simulink model "untitled5"  (R2019b)
settings: Solver=VariableStepAuto  StartTime=0.0  StopTime=60  RelTol=1e-3
model workspace (MAT data in the model file):
  A = Simulink.Signal
  A.DataType = 'double'
  A.Min = 0
  A.Dimensions = 1
  A.DimensionsMode = 'auto'
  A.Complexity = 'auto'
  A.SampleTime = -1
  A.SamplingMode = 'auto'
  A.InitialValue = '0'
values from neighbouring files (symbols this model uses):
  Brad = 0.17    [lab5.m]
  J = 0.0023    [lab5.m]
  Ke = Km    (= 0.29)    [lab5.m]
  Km = 0.29    [lab5.m]
  Kr = 70    [lab5.m]
  Ks = 250    [lab5.m]
  L = 0.0047    [lab5.m]
  R = 4.7    [lab5.m]
  Rad = 0.0275    [lab5.m]
  Um = 3.5    [lab5.m]
settings Model: Creator=Ivan  LastModifiedBy=Ivan
settings SolverCC: AlgebraicLoopSolver=LineSearch

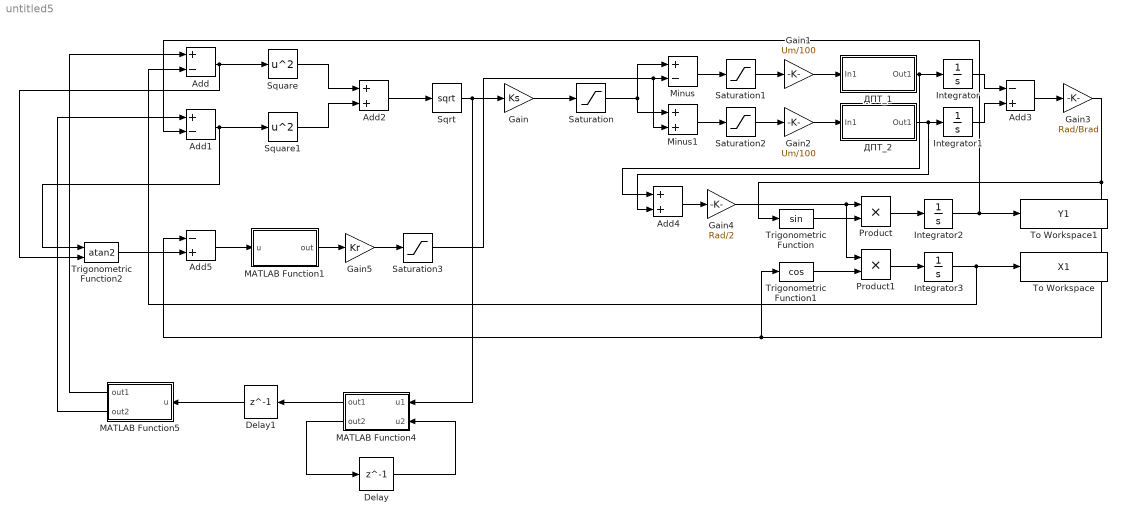
== system untitled5 ==
  Add : Sum  Inputs=+-
  Add1 : Sum  Inputs=+-
  Add2 : Sum
  Add3 : Sum  Inputs=-+
  Add4 : Sum
  Add5 : Sum  Inputs=-+
  Delay : Delay  DelayLength=1  InitialCondition=0
  Delay1 : Delay  DelayLength=1  InitialCondition=0
  Gain : Gain  Gain=Ks
  Gain1 : Gain  Gain=Um/100
  Gain2 : Gain  Gain=Um/100
  Gain3 : Gain  Gain=Rad/Brad
  Gain4 : Gain  Gain=Rad/2
  Gain5 : Gain  Gain=Kr
  Integrator{,1..3} (4 alike) : Integrator
  MATLAB Function1 : MATLAB Function  TreatAsAtomicUnit=on  VariantControl=Variant1
  MATLAB Function4 : MATLAB Function  TreatAsAtomicUnit=on  VariantControl=Variant1
  MATLAB Function5 : MATLAB Function  TreatAsAtomicUnit=on  VariantControl=Variant1
  Minus : Sum  Inputs=+-
  Minus1 : Sum
  Product : Product
  Product1 : Product
  Saturation : Saturate  UpperLimit=80  LowerLimit=-80
  Saturation1 : Saturate  UpperLimit=100  LowerLimit=-100
  Saturation2 : Saturate  UpperLimit=100  LowerLimit=-100
  Saturation3 : Saturate  UpperLimit=20  LowerLimit=-20
  Sqrt : Sqrt  SaturateOnIntegerOverflow=on
  Square : Math  Operator=square  SignedPower=off  SaturateOnIntegerOverflow=on
  Square1 : Math  Operator=square  SignedPower=off  SaturateOnIntegerOverflow=on
  To Workspace : ToWorkspace  VariableName=X1  SaveFormat=Timeseries  SampleTime=-1
  To Workspace1 : ToWorkspace  VariableName=Y1  SaveFormat=Timeseries  SampleTime=-1
  Trigonometric Function : Trigonometry
  Trigonometric Function1 : Trigonometry  Operator=cos
  Trigonometric Function2 : Trigonometry  Operator=atan2
  "ДПТ_1 " : Subsystem
  "ДПТ_2 " : Subsystem
  wires:
  Add/1 -> Trigonometric Function2/2, Square/1
  Add1/1 -> Trigonometric Function2/1, Square1/1
  Square/1 -> Add2/1
  Square1/1 -> Add2/2
  Add2/1 -> Sqrt/1
  Sqrt/1 -> MATLAB Function4/1(u1), Gain/1
  Gain/1 -> Saturation/1
  Saturation/1 -> Minus/1, Minus1/1
  Minus/1 -> Saturation1/1
  Minus1/1 -> Saturation2/1
  Saturation1/1 -> Gain1/1
  Saturation2/1 -> Gain2/1
  Gain1/1 -> "ДПТ_1 "/1(In1)
  Gain2/1 -> "ДПТ_2 "/1(In1)
  "ДПТ_1 "/1(Out1) -> Add4/1, Integrator/1
  "ДПТ_2 "/1(Out1) -> Add4/2, Integrator1/1
  Integrator/1 -> Add3/1
  Integrator1/1 -> Add3/2
  Add3/1 -> Gain3/1
  Add4/1 -> Gain4/1
  Gain4/1 -> Product1/1, Product/1
  Gain3/1 -> Trigonometric Function/1, Trigonometric Function1/1, Add5/1
  Trigonometric Function/1 -> Product/2
  Trigonometric Function1/1 -> Product1/2
  Product/1 -> Integrator2/1
  Product1/1 -> Integrator3/1
  Trigonometric Function2/1 -> Add5/2
  Gain5/1 -> Saturation3/1
  Saturation3/1 -> Minus1/2, Minus/2
  Integrator2/1 -> To Workspace1/1, Add1/2
  Integrator3/1 -> To Workspace/1, Add/2
  Add5/1 -> MATLAB Function1/1(u)
  MATLAB Function1/1(out) -> Gain5/1
  MATLAB Function5/1(out1) -> Add/1
  MATLAB Function5/2(out2) -> Add1/1
  MATLAB Function4/1(out1) -> Delay1/1
  Delay/1 -> MATLAB Function4/2(u2)
  MATLAB Function4/2(out2) -> Delay/1
  Delay1/1 -> MATLAB Function5/1(u)

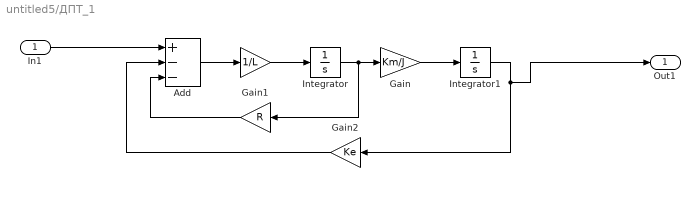
== system untitled5/ДПТ_1  ==
  In1 : Inport
  " " : Gain  Gain=1/L
  Add : Sum  Inputs=+--
  Gain : Gain  Gain=Km/J
  Gain1 : Gain  Gain=R
  Gain2 : Gain  Gain=Ke
  Integrator : Integrator
  Integrator1 : Integrator
  Out1 : Outport
  wires:
  In1/1 -> Add/1
  Add/1 -> " "/1
  " "/1 -> Integrator/1
  Integrator/1 -> Gain1/1, Gain/1
  Gain/1 -> Integrator1/1
  Integrator1/1 -> Out1/1, Gain2/1
  Gain1/1 -> Add/3
  Gain2/1 -> Add/2

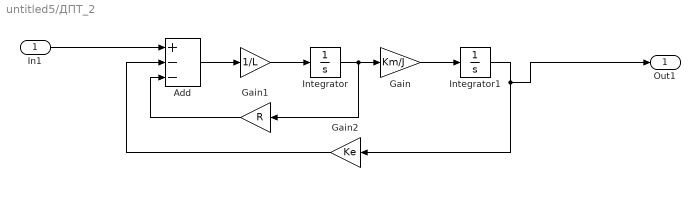
== system untitled5/ДПТ_2  ==
  In1 : Inport
  " " : Gain  Gain=1/L
  Add : Sum  Inputs=+--
  Gain : Gain  Gain=Km/J
  Gain1 : Gain  Gain=R
  Gain2 : Gain  Gain=Ke
  Integrator : Integrator
  Integrator1 : Integrator
  Out1 : Outport
  wires:
  In1/1 -> Add/1
  Add/1 -> " "/1
  " "/1 -> Integrator/1
  Integrator/1 -> Gain1/1, Gain/1
  Gain/1 -> Integrator1/1
  Integrator1/1 -> Out1/1, Gain2/1
  Gain1/1 -> Add/3
  Gain2/1 -> Add/2

== matlab function untitled5/MATLAB Function1 ==
  data: u input; out output
function out = fcn(u)
%%codegen
    if (abs(u)>3.14)
        y=u-sign(u)*2*3.14;
    else
        y=u;
    end
out = y;

== matlab function untitled5/MATLAB Function4 ==
  data: u1 input; out1 output; u2 input; out2 output
function [out1,out2] = fcn(u1,u2)
%%codegen
    j = u2;
    if (u1 <= 0.05)
        j = j + 1;
    end
out1 = j;out2 = j;

== matlab function untitled5/MATLAB Function5 ==
  data: u input; out1 output; out2 output
function [out1,out2] = fcn(u)
%%codegen
    x=1;y=1;
    switch (u)
        case 0
            x = 1;
            y = 1;
        case 1
            x = 1;
            y = -1;
        case 2
            x = -1;
            y = -1;
        case 3
            x = -1;
            y = 1;
        case 4
            x = 1;
            y = 1;
        otherwise
            x = 1;
            y = 1;
    end
        
out1 = x; out2 = y;
